simulink model "Self_Made_VCO"  (R2019b)
settings: Solver=VariableStepAuto  StartTime=0.0  StopTime=0.00005  RelTol=1e-3
libraries: impairlib x1
settings Model: Creator=connerhannon  LastModifiedBy=connerhannon
settings SolverCC: MaxConsecutiveZCs=1  MaxConsecutiveMinStep=100000

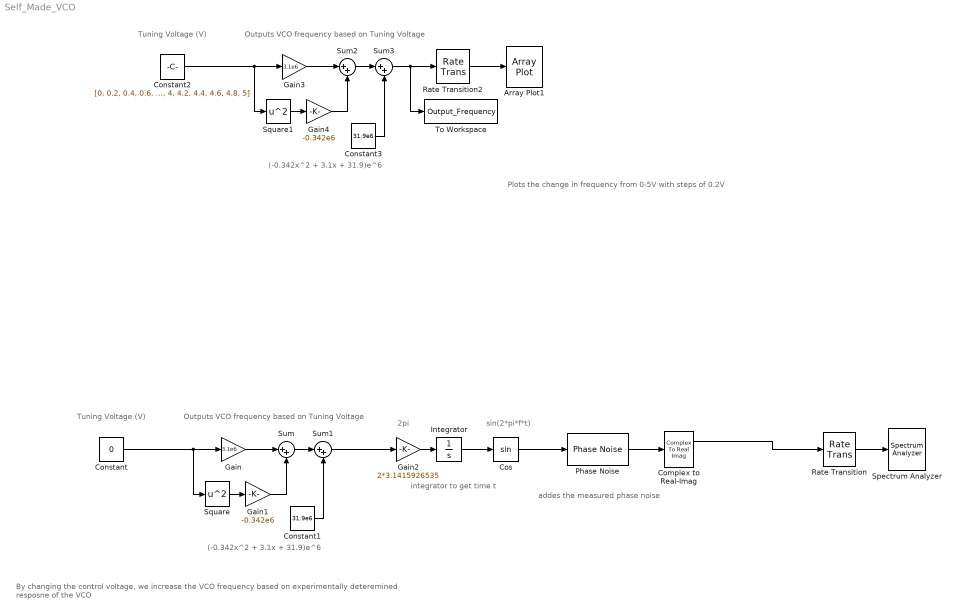
== system Self_Made_VCO ==
  note: Plots the change in frequency from 0-5V
      | with steps of 0.2V
  note: Outputs VCO frequency based on Tuning Voltage
  note: addes the measured phase noise
  note: (-0.342x^2 + 3.1x + 31.9)e^6
  note: By changing the control voltage, we increase the VCO frequency based on experimentally deteremined resposne of the VCO
  note: sin(2*pi*f*t)
  note: integrator to get time t
  note: 2pi
  note: Tuning Voltage
      | (V)
  note: Tuning Voltage
      | (V)
  note: (-0.342x^2 + 3.1x + 31.9)e^6
  note: Outputs VCO frequency based on Tuning Voltage
  Array Plot1 : ArrayPlot
  Complex to Real-Imag : ComplexToRealImag
  Constant : Constant  Value=0  OutMin=[0]  OutMax=[5]
  Constant1 : Constant  Value=31.9e6
  Constant2 : Constant  Value=[0, 0.2, 0.4, 0.6, 0.8, 1, 1.2, 1.4, 1.6, 1.8, 2, 2.2, 2.4, 2.6, 2.8, 3, 3.2, 3.4, 3.6, 3.8, 4, 4.2, 4.4, 4.6, 4.8, 5]  OutMin=[0]  OutMax=[5]
  Constant3 : Constant  Value=31.9e6
  Cos : Trigonometry  OutputSignalType=complex
  Gain : Gain  Gain=3.1e6
  Gain1 : Gain  Gain=-0.342e6
  Gain2 : Gain  Gain=2*3.1415926535
  Gain3 : Gain  Gain=3.1e6
  Gain4 : Gain  Gain=-0.342e6
  Integrator : Integrator
  Phase Noise : impairlib/Phase Noise  Level=[ -36, -73, -83, -90, -112 ]  FrequencyOffset=[ 100, 400, 1000, 5000, 250000]  SampleRate=550000  RandomStream=mt19937ar with seed  Seed=1e6  SimulateUsing=Interpreted execution
      settings: SourceProductName=SerDes Toolbox  SourceProductBaseCode=SX
  Rate Transition : RateTransition  OutPortSampleTime=1/1000000000
  Rate Transition2 : RateTransition  OutPortSampleTime=1/1000000000
  Spectrum Analyzer : SpectrumAnalyzer
  Square : Math  Operator=square  SignedPower=off  SaturateOnIntegerOverflow=on
  Square1 : Math  Operator=square  SignedPower=off  SaturateOnIntegerOverflow=on
  Sum{,1..3} (4 alike) : Sum  Inputs=|++
  To Workspace : ToWorkspace  VariableName=Output_Frequency  SaveFormat=Timeseries  SampleTime=-1
  wires:
  Gain/1 -> Sum/1
  Constant/1 -> Gain/1, Square/1
  Gain2/1 -> Integrator/1
  Integrator/1 -> Cos/1
  Cos/1 -> Phase Noise/1
  Rate Transition/1 -> Spectrum Analyzer/1
  Sum/1 -> Sum1/1
  Sum1/1 -> Gain2/1
  Constant1/1 -> Sum1/2
  Gain1/1 -> Sum/2
  Square/1 -> Gain1/1
  Constant3/1 -> Sum3/2
  Gain3/1 -> Sum2/1
  Sum2/1 -> Sum3/1
  Gain4/1 -> Sum2/2
  Square1/1 -> Gain4/1
  Constant2/1 -> Gain3/1, Square1/1
  Rate Transition2/1 -> Array Plot1/1
  Sum3/1 -> To Workspace/1, Rate Transition2/1
  Phase Noise/1 -> Complex to Real-Imag/1
  Complex to Real-Imag/1 -> Rate Transition/1
